simulink model "Demo"  (Simulink 9.2)
settings: Solver=FixedStepDiscrete  StartTime=0.0  StopTime=10.0  FixedStep=1  RelTol=1e-3  EnableMultiTasking=on
PreLoadFcn:
  | DataStore = Simulink.Signal;
  | DataStore.Description = 'Stores data for demo.';
  | DataStore.DataType = 'uint16';
  | DataStore.Complexity = 'real';
  | DataStore.Dimensions = 1;
  | DataStore.SamplingMode='Sample based';
  | DataStore.SampleTime = 1;
settings Model: Creator=monika  LastModifiedBy=monika  ExtModeAutoUpdateStatusClock=off
settings DataIOCC: SaveFormat=StructureWithTime  SignalLoggingSaveFormat=Dataset
settings OptimizationCC: BlockReduction=off  BooleanDataType=off  ExpressionDepthLimit=2147483647  InitFltsAndDblsToZero=on
settings DebuggingCC: SaveWithParameterizedLinksMsg=none  UnderspecifiedInitializationDetection=Simplified  MergeDetectMultiDrivingBlocksExec=error  SignalResolutionControl=TryResolveAllWithWarning  MultiTaskDSMMsg=warning  MultiTaskCondExecSysMsg=none
settings HardwareCC: TargetUnknown=on
settings GRTTargetCC: TargetFcnLib=ansi_tfl_tmw.mat
settings ConfigComp: CovMetricSettings=d

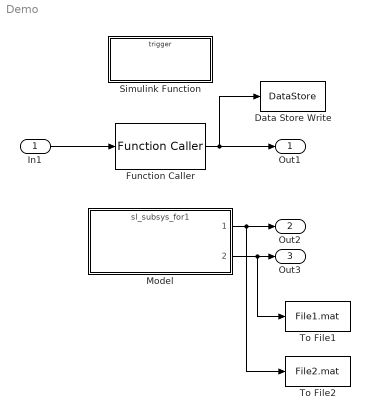
== system Demo ==
  In1 : Inport  OutDataTypeStr=uint16  PortDimensions=1  SampleTime=1
  Data Store Write : DataStoreWrite  DataStoreName=DataStore  SampleTime=1
  Function Caller : FunctionCaller  FunctionPrototype=y = f(u)  InputArgumentSpecifications=uint16(1)  OutputArgumentSpecifications=uint16(1)
  Model : ModelReference  ModelNameDialog=sl_subsys_for1  SimulationMode=Normal  ModelReferenceVersion=1.66
  Simulink Function : Subsystem  TreatAsAtomicUnit=on
  To File1 : ToFile  Filename=File1.mat  MatrixName=Out3  SaveFormat=Timeseries
  To File2 : ToFile  Filename=File2.mat  MatrixName=Out2  SaveFormat=Timeseries
  Out1 : Outport  PortDimensions=1
  Out2 : Outport  Port=2
  Out3 : Outport  Port=3
  wires:
  In1/1 -> Function Caller/1
  Model/2 -> To File1/1, Out3/1
  Model/1 -> To File2/1, Out2/1
  Function Caller/1 -> Data Store Write/1, Out1/1

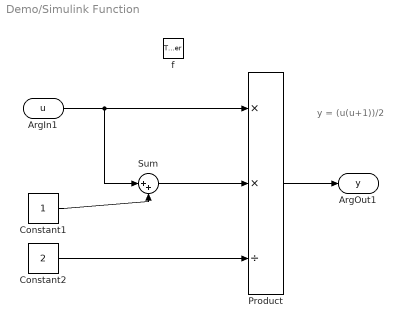
== system Demo/Simulink Function ==
  note: y = (u(u+1))/2
  f : TriggerPort  TriggerType=function-call  IsSimulinkFunction=on  FunctionName=f  VariantControl=(inherit)
  Constant1 : Constant  OutDataTypeStr=uint16
  Constant2 : Constant  Value=2  OutDataTypeStr=uint16
  Product : Product  Inputs=**/  OutDataTypeStr=uint16
  Sum : Sum  Inputs=|++
  ArgIn1 : ArgIn  DisableCoverage=on  OutDataTypeStr=uint16  ArgumentName=u
  ArgOut1 : ArgOut  DisableCoverage=on  OutDataTypeStr=uint16  ArgumentName=y
  wires:
  Product/1 -> ArgOut1/1
  Constant2/1 -> Product/3
  Sum/1 -> Product/2
  ArgIn1/1 -> Sum/1, Product/1
  Constant1/1 -> Sum/2
